simulink model "ejercicio_3_05_10_jevg"  (R2021a)
settings: Solver=VariableStepAuto  StartTime=0.0  StopTime=10  RelTol=1e-3
libraries: fl_lib x9, nesl_utility x4
settings Model: LastModifiedBy=user
settings DebuggingCC: UnconnectedInputMsg=none  UnconnectedOutputMsg=none  UnconnectedLineMsg=none
settings ModelReferenceCC: EnableRefExpFcnMdlSchedulingChecks=off
settings RTWCC: Description=Generic Real-Time Target  DLArmComputeVersion=20.02.1

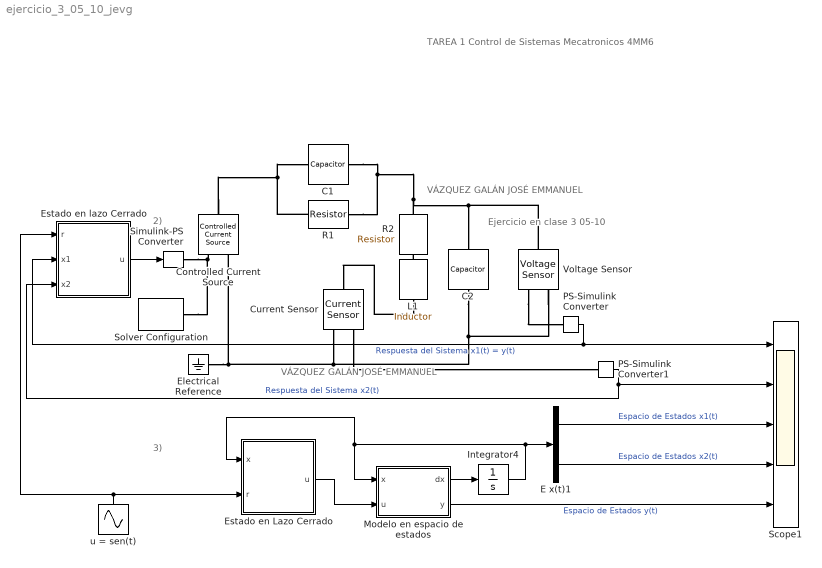
== system ejercicio_3_05_10_jevg ==
  note: TAREA 1
      | Control de Sistemas Mecatronicos 4MM6
  note: VÁZQUEZ GALÁN JOSÉ EMMANUEL
  note: 3)
  note: 2)
  note: Ejercicio en clase 3
      | 05-10
  note: VÁZQUEZ GALÁN JOSÉ EMMANUEL
  C1 : fl_lib/Electrical/Electrical Elements/Capacitor  c=1 F  r=1e-6 Ohm  g=0 1/Ohm  i_specify=off  i_priority=None  i=0 A  i_nominal_specify=off  i_nominal_unit=A  i_nominal_value=1  v_specify=off  v_priority=None  v=0 V  v_nominal_specify=off  v_nominal_unit=V  v_nominal_value=1  vc_specify=off  vc_priority=High  vc=0 V  vc_nominal_specify=off  vc_nominal_unit=V  vc_nominal_value=1
  C2 : fl_lib/Electrical/Electrical Elements/Capacitor  c=1 F  r=1e-6 Ohm  g=0 1/Ohm  i_specify=off  i_priority=None  i=0 A  i_nominal_specify=off  i_nominal_unit=A  i_nominal_value=1  v_specify=off  v_priority=None  v=0 V  v_nominal_specify=off  v_nominal_unit=V  v_nominal_value=1  vc_specify=off  vc_priority=High  vc=0 V  vc_nominal_specify=off  vc_nominal_unit=V  vc_nominal_value=1
  Controlled Current Source : fl_lib/Electrical/Electrical Sources/Controlled Current Source
  Current Sensor : fl_lib/Electrical/Electrical Sensors/Current Sensor
  E x(t)1 : Demux  Outputs=2
  Electrical Reference : fl_lib/Electrical/Electrical Elements/Electrical Reference
  Estado en Lazo Cerrado : MATLAB Function  TreatAsAtomicUnit=on
  Estado en lazo Cerrado : MATLAB Function  TreatAsAtomicUnit=on
  Integrator4 : Integrator  InitialCondition=[0;0]
  L1 : fl_lib/Electrical/Electrical Elements/Inductor  l=1 H  r=0 Ohm  g=1e-9 1/Ohm  i_specify=off  i_priority=None  i=0 A  i_nominal_specify=off  i_nominal_unit=A  i_nominal_value=1  v_specify=off  v_priority=None  v=0 V  v_nominal_specify=off  v_nominal_unit=V  v_nominal_value=1  i_L_specify=off  i_L_priority=High  i_L=0 A  i_L_nominal_specify=off  i_L_nominal_unit=A  i_L_nominal_value=1
  Modelo en espacio de estados : MATLAB Function  TreatAsAtomicUnit=on
  PS-Simulink Converter : nesl_utility/PS-Simulink Converter  PhysicalDomain=network_engine_domain  SubClassName=ps_output  LeftPortType=input  RightPortType=output  PseudoPeriodic=off  Frequencies=[]  Unit=inherit  AffineConversion=off
      settings: SourceProductBaseCode=PW,SS
  PS-Simulink Converter1 : nesl_utility/PS-Simulink Converter  PhysicalDomain=network_engine_domain  SubClassName=ps_output  LeftPortType=input  RightPortType=output  PseudoPeriodic=off  Frequencies=[]  Unit=inherit  AffineConversion=off
      settings: SourceProductBaseCode=PW,SS
  R1 : fl_lib/Electrical/Electrical Elements/Resistor  R=1 Ohm  i_specify=off  i_priority=None  i=0 A  i_nominal_specify=off  i_nominal_unit=A  i_nominal_value=1  v_specify=off  v_priority=None  v=0 V  v_nominal_specify=off  v_nominal_unit=V  v_nominal_value=1
  R2 : fl_lib/Electrical/Electrical Elements/Resistor  R=1 Ohm  i_specify=off  i_priority=None  i=0 A  i_nominal_specify=off  i_nominal_unit=A  i_nominal_value=1  v_specify=off  v_priority=None  v=0 V  v_nominal_specify=off  v_nominal_unit=V  v_nominal_value=1
  Scope1 : Scope  NumInputPorts=5
  Simulink-PS Converter : nesl_utility/Simulink-PS Converter  PhysicalDomain=network_engine_domain  SubClassName=ps_input  LeftPortType=input  RightPortType=output  PseudoPeriodic=off  Frequencies=[]  NoiseDistribution=none  NoiseParameters=[]  Unit=1  AffineConversion=off  FilteringAndDerivatives=provide  SimscapeFilterOrder=1  InputFilterTimeConstant=0.001  UdotUserProvided=0
      settings: SourceProductBaseCode=PW,SS
  Solver Configuration : nesl_utility/Solver Configuration  PhysicalDomain=network_engine_domain  SubClassName=solver  LeftPortType=input  RightPortType=generic  Tones=[]  Harmonics=[]  SimulateNoise=off  Profile=off  UseLocalSampling=off  EnableSwitchedLinearOptims=on  FrequencyDomain=off  UseCCode=off  RelTol=0.001  AbsTol=0.001  MinStep=1e-09  ToWorkspace=off  RevertToSquareIcSolve=off  NumHomotopyIterations=100  PhasorMode=off  PhasorModeNumHarmonics=1  DoDC=on  ResidualTolerance=1e-09  UseLocalSolver=off  LocalSolverChoice=NE_BACKWARD_EULER_ADVANCER  LocalSolverSampleTime=0.001  DoFixedCost=off  MaxNonlinIter=3  MaxModeIter=2  ComputeImpulses=off  ImpulseIterations=2  LinearAlgebra=auto  EquationFormulation=NE_TIME_EF  DelaysMemoryBudget=1024  AutomaticFiltering=on  FilteringTimeConstant=0.001  PartitionStorageMethod=AS_NEEDED  PartitionMemoryBudget=1024  PartitionMethod=ROBUST
      settings: SourceProductBaseCode=PW,SS
  Voltage Sensor : fl_lib/Electrical/Electrical Sensors/Voltage Sensor
  "u = sen(t) " : Sin  SampleTime=0
  wires:
  E x(t)1/1 -> Scope1/3  "Espacio de Estados x1(t)"
  Modelo en espacio de estados/1(dx) -> Integrator4/1
  Integrator4/1 -> E x(t)1/1, Modelo en espacio de estados/1(x), Estado en Lazo Cerrado/1(x)
  E x(t)1/2 -> Scope1/4  "Espacio de Estados x2(t)"
  Modelo en espacio de estados/2(y) -> Scope1/5  "Espacio de Estados y(t)"
  PS-Simulink Converter/1 -> Scope1/1, Estado en lazo Cerrado/2(x1)  "Respuesta del Sistema x1(t) = y(t)"
  PS-Simulink Converter1/1 -> Estado en lazo Cerrado/3(x2), Scope1/2  "Respuesta del Sistema x2(t)"
  Estado en Lazo Cerrado/1(u) -> Modelo en espacio de estados/2(u)
  "u = sen(t) "/1 -> Estado en Lazo Cerrado/2(r), Estado en lazo Cerrado/1(r)
  Estado en lazo Cerrado/1(u) -> Simulink-PS Converter/1
  connections:
  R2/LConn1 -- C1/RConn1 -- R1/RConn1 -- Voltage Sensor/LConn1 -- C2/LConn1
  L1/LConn1 -- R2/RConn1
  R1/LConn1 -- Controlled Current Source/LConn1 -- C1/LConn1
  L1/RConn1 -- Current Sensor/LConn1
  Voltage Sensor/RConn1 -- PS-Simulink Converter/LConn1
  Simulink-PS Converter/RConn1 -- Solver Configuration/RConn1 -- Controlled Current Source/RConn1
  C2/RConn1 -- Current Sensor/RConn2 -- Electrical Reference/LConn1 -- Controlled Current Source/RConn2 -- Voltage Sensor/RConn2
  Current Sensor/RConn1 -- PS-Simulink Converter1/LConn1

== matlab function ejercicio_3_05_10_jevg/Estado en lazo Cerrado ==
  data: r input; u output; x1 input; x2 input
function u = fcn(r,x1,x2)
% Esta función calcula el control u basado en la entrada r y el estado actual del sistema x.

% Definiendo la matriz de ganancias K
K = [3 0];

% Organizando las variables de estado en un vector columna
x = [x1,x2]';

% Calculando la señal de control u usando la retroalimentación de estado
u = r - K*x;

== matlab function ejercicio_3_05_10_jevg/Estado en Lazo Cerrado ==
  data: x input; r input; u output
function u = fcn(x,r)
% Esta función calcula el control u basado en la entrada r y el estado actual del sistema x (como vector).

% Definiendo la matriz de ganancias K
K = [3 0];

% Calculando la señal de control u usando la retroalimentación de estado
u = r - K*x;

== matlab function ejercicio_3_05_10_jevg/Modelo en espacio de estados ==
  data: x input; dx output; u input; y output
function [dx,y] = fcn(x,u)
% Esta función calcula la derivada del estado dx y la salida y basado en el estado actual x y la señal de control u.
% Definiendo la matriz A del sistema en el espacio de estados
A = [0 -1; 
     1 -1];
% Definiendo la matriz B del sistema en el espacio de estados
B = [1; 
    0];

% Definiendo la matriz C para la salida
C=[1 0];

% Calculando la derivada del estado
dx = A*x + B*u;

% Calculando la salida
y = C*x;
